simulink model "dspsinecomp"  (Simulink 4.00)
settings: Solver=FixedStepDiscrete  StartTime=0.0  StopTime=inf  RelTol=1e-3
libraries: dspsrcs3 x4, dspstat3 x1
Description:
  | Comparison of sine wave generation techniques.
settings Model: CovMetricSettings=d  Creator=don  LastModifiedBy=ashah  SaveTime=off  SaveOutput=off  LimitDataPoints=off  SingleTaskRateTransMsg=error  IntegerOverflowMsg=none  RTWOptions=-aRollThreshold=2  ExtModeTrigMode=oneshot  ExtModeArmWhenConnect=off  BlockReductionOpt=off

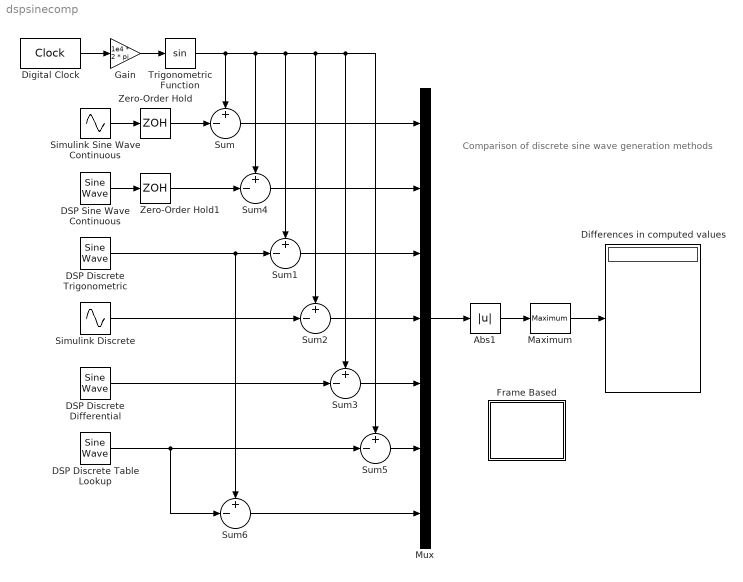
== system dspsinecomp ==
  note: Comparison of discrete
      | sine wave generation methods
  Abs1 : Abs  SaturateOnIntegerOverflow=on
  DSP Discrete Differential : dspsrcs3/Sine Wave  Amplitude=1  Frequency=1e4  Phase=0  SampleMode=Discrete  OutComplex=Real  CompMethod=Differential  TableSize=Speed  SampleTime=1e-5  SamplesPerFrame=1  ResetState=Restart at time zero
  DSP Discrete Table Lookup : dspsrcs3/Sine Wave  Amplitude=1  Frequency=1e4  Phase=0  SampleMode=Discrete  OutComplex=Real  CompMethod=Table Lookup  TableSize=Speed  SampleTime=1e-5  SamplesPerFrame=1  ResetState=Restart at time zero
  DSP Discrete Trigonometric : dspsrcs3/Sine Wave  Amplitude=1  Frequency=1e4  Phase=0  SampleMode=Discrete  OutComplex=Real  CompMethod=Trigonometric Fcn  TableSize=Speed  SampleTime=1e-5  SamplesPerFrame=1  ResetState=Restart at time zero
  DSP Sine Wave Continuous : dspsrcs3/Sine Wave  Amplitude=1  Frequency=1e4  Phase=0  SampleMode=Continuous  OutComplex=Real  CompMethod=Trigonometric Fcn  TableSize=Speed  SampleTime=1/1000  SamplesPerFrame=1  ResetState=Restart at time zero
  Differences in computed values : Display
      settings: Format=short
  Digital Clock : DigitalClock  SampleTime=1e-5
  Frame Based : Subsystem
      settings: OpenFcn=dspfsinecomp;  RTWFcnNameOpts=Auto  RTWFileNameOpts=Auto
      mask Display: disp('Frame-based\nVersion')
  Gain : Gain  Gain=1e4 * 2 * pi  Multiplication=Element-wise(K.*u)  SaturateOnIntegerOverflow=on
  Maximum : dspstat3/Maximum  fcn=Running  reset=None
  Mux : Mux  Inputs=7  BusCreatorMode=off
  Simulink Discrete : Sin  SineType=Time-based  Amplitude=1  Bias=0  Frequency="1e4  * 2 * pi"  Phase=0  Samples=10  SampleTime=1e-5  Offset=0
  Simulink Sine Wave Continuous : Sin  SineType=Time-based  Amplitude=1  Bias=0  Frequency=1e4 * 2 * pi  Phase=0  Samples=10  SampleTime=0  Offset=0
  Sum{,1..6} (7 alike) : Sum  Inputs=+-|  SaturateOnIntegerOverflow=on
  Trigonometric Function : Trigonometry  Operator=sin  OutputSignalType=auto
  Zero-Order Hold : ZeroOrderHold  SampleTime=1e-5
  Zero-Order Hold1 : ZeroOrderHold  SampleTime=1e-5
  wires:
  Gain/1 -> Trigonometric Function/1
  Digital Clock/1 -> Gain/1
  Trigonometric Function/1 -> Sum/1, Sum1/1, Sum2/1, Sum3/1, Sum5/1, Sum4/1
  Sum5/1 -> Mux/6
  Sum6/1 -> Mux/7
  DSP Discrete Table Lookup/1 -> Sum5/2, Sum6/2
  Sum3/1 -> Mux/5
  DSP Discrete Differential/1 -> Sum3/2
  Sum2/1 -> Mux/4
  Simulink Discrete/1 -> Sum2/2
  Sum1/1 -> Mux/3
  DSP Discrete Trigonometric/1 -> Sum1/2, Sum6/1
  DSP Sine Wave Continuous/1 -> Zero-Order Hold1/1
  Zero-Order Hold1/1 -> Sum4/2
  Sum4/1 -> Mux/2
  Simulink Sine Wave Continuous/1 -> Zero-Order Hold/1
  Zero-Order Hold/1 -> Sum/2
  Sum/1 -> Mux/1
  Mux/1 -> Abs1/1
  Abs1/1 -> Maximum/1
  Maximum/1 -> Differences in computed values/1

== system dspsinecomp/Frame Based ==
